simulink model "WTLV"  (R2023a)
settings: Solver=VariableStepAuto  StartTime=0.0  StopTime=5  RelTol=1e-3
values from neighbouring files (symbols this model uses):
  Cbus = 80e-3    (= 0.08)    [DFIG_init5.m]
  D = 1e-3    (= 0.001)    [DFIG_init5.m]
  f = 50    [DFIG_init5.m]
  Fs = Vs*sqrt(2/3)/(2*pi*f)    [DFIG_init5.m]
  fsw = 4e3    (= 4000)    [DFIG_init5.m]
  Is = 1760    [DFIG_init5.m]
  J = 127    [DFIG_init5.m]
  ki_id = (wni^2)*Lr*sigma    (= 491.599501999)    [DFIG_init5.m]
  ki_idg = (wnig^2)*Lg    (= 56.8489213503)    [DFIG_init5.m]
  ki_iq = ki_id    (= 491.599501999)    [DFIG_init5.m]
  ki_iqg = ki_idg    (= 56.8489213503)    [DFIG_init5.m]
  ki_n = (wnn^2)*J/p    (= 25400)    [DFIG_init5.m]
  ki_v = -300000    [DFIG_init5.m]
  Kopt = ((0.5*ro*pi* (Radio^5) *Cp_max)/(lambda_opt^3))    (= 296454.198186)    [DFIG_init5.m]
  kp_id = (2*wni*sigma*Lr)-Rr    (= 0.5771)    [DFIG_init5.m]
  kp_idg = (2*wnig*Lg)-Rg    (= 0.301572894745)    [DFIG_init5.m]
  kp_iq = kp_id    (= 0.5771)    [DFIG_init5.m]
  kp_iqg = kp_idg    (= 0.301572894745)    [DFIG_init5.m]
  kp_n = (2*wnn*J)/p    (= 2540)    [DFIG_init5.m]
  kp_v = -1000    [DFIG_init5.m]
  Kpg = 1/(1.5*Vs*sqrt(2/3))    [DFIG_init5.m]
  Kqg = -Kpg    [DFIG_init5.m]
  kT = -1.5*p*(Lm/Ls)*Fs    [DFIG_init5.m]
  Lg = 400e-6    (= 0.0004)    [DFIG_init5.m]
  Lm = 2.5e-3    (= 0.0025)    [DFIG_init5.m]
  Lr = Lm + Lsi    (= 0.002587)    [DFIG_init5.m]
  Ls = Lm + Lsi    (= 0.002587)    [DFIG_init5.m]
  Lsi = 0.087e-3    (= 8.7e-05)    [DFIG_init5.m]
  N = 100    [DFIG_init5.m]
  p = 2    [DFIG_init5.m]
  Ps = 2e6    (= 2000000)    [DFIG_init5.m]
  Radio = 42    [DFIG_init5.m]
  Rcrowbar = 0.2    [DFIG_init5.m]
  Rg = 20e-6    (= 2e-05)    [DFIG_init5.m]
  ro = 1.225    [DFIG_init5.m]
  Rr = 2.9e-3    (= 0.0029)    [DFIG_init5.m]
  Rs = 2.6e-3    (= 0.0026)    [DFIG_init5.m]
  sigma = 1-Lm^2/(Ls*Lr)    (= 0.0661284179513)    [DFIG_init5.m]
  smax = 1/3    (= 0.333333333333)    [DFIG_init5.m]
  t_dip = 3    [DFIG_init5.m]
  t_normal = 4.17    [DFIG_init5.m]
  t_recover = 3.5    [DFIG_init5.m]
  tab_lambda = [0.1:0.01:11.8]    [DFIG_init5.m]
  Tcrowbar = 0.1    [DFIG_init5.m]
  Tem = 12732    [DFIG_init5.m]
  Ts = 1/fsw/50    (= 5e-06)    [DFIG_init5.m]
  Vbus = 1150    [DFIG_init5.m]
  Vs = 690    [DFIG_init5.m]
undefined symbols (not defined in the file or in its folder): Ct, DiscIntNeverNeededParam
libraries: spsSeriesRLCBranchLib x5, spsUniversalBridgeLib x3, spsThreePhaseVIMeasurementLib x3, spsPWMGenerator2LevelLib x2, spsAsynchronousMachineSIUnitsLib x1, spsGroundLib x1, spsIdealSwitchLib x1, spsThreePhaseProgrammableVoltageSourceLib x1, spsThreePhaseTransformerTwoWindingsLib x1, spsEdgeDetectorLib x1, eeGeneralControl x1, sps_lib x1
settings Model: SimulationMode=accelerator  Creator=Qingyuan  LastModifiedBy=User
settings OptimizationCC: ReuseModelBlockBuffer=off

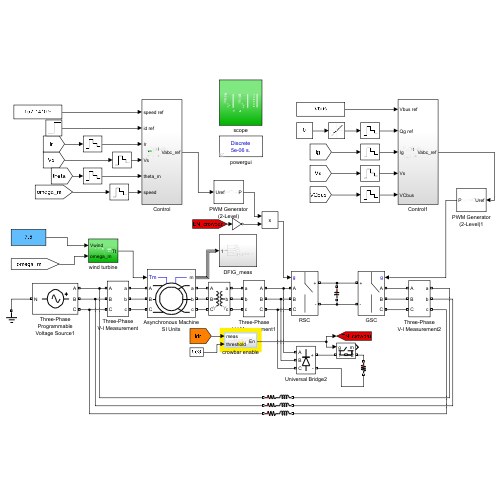
[thumbnail: Simulink's stored preview of the top-level diagram]
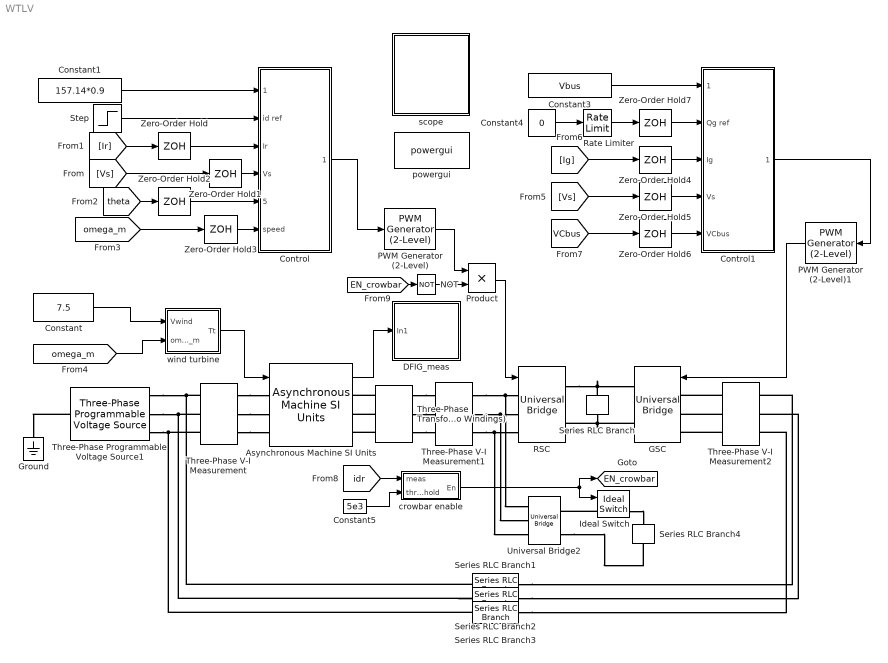
== system WTLV ==
  Asynchronous Machine SI Units : spsAsynchronousMachineSIUnitsLib/Asynchronous Machine SI Units  RotorType=Wound  PresetModel=No  MechanicalLoad=Torque Tm  ShowDetailedParameters=on  ReferenceFrame=Rotor  Units=SI  MeasurementBus=off  NominalParameters=[Ps Vs f]  VoltageRatio=1  Stator=[Rs Lsi]  Rotor=[Rr Lsi]  Cage1=[0.4155 0.002066]  Cage2=[0.4168 0.0003495]  Lm=Lm  Mechanical=[J D p]  PolePairs=2  InitialConditions=[1 0 0 0 0 0 0 0]  SimulateSaturation=off  Saturation=[14.03593122, 27.81365428, 53.79336849, 72.68890987, 97.98006896, 148.6815601, 215.7428561, 302.9841135, 428.7778367 ; 230, 322, 414, 460, 506, 552, 598, 644, 690]  LoadFlowParameters=1492000  TsPowergui=0  TsBlock=-1  IterativeModel=Trapezoidal non iterative  IterativeDiscreteModel=Trapezoidal non iterative  Pmec=1.4e6
  Constant : Constant  Value=7.5
  Constant1 : Constant  Value=157.14*0.9
  Constant3 : Constant  Value=Vbus
  Constant4 : Constant  Value=0
  Constant5 : Constant  Value=5e3
  Control : Subsystem
  Control1 : Subsystem
  DFIG_meas : Subsystem
  GSC : spsUniversalBridgeLib/Universal Bridge  Arms=3  SnubberResistance=1e5  SnubberCapacitance=inf  Device=Ideal Switches  Ron=1e-3  Lon=0  ForwardVoltages="[  0  0  ]"  ForwardVoltage=0  GTOparameters=[ 10e-6 , 20e-6 ]  IGBTparameters=[ 1e-6 , 2e-6 ]  Measurements=None  Measurements_2=None  converterType=Rectifier
  Ground : spsGroundLib/Ground  LConnTagsString=a
  Ideal Switch : spsIdealSwitchLib/Ideal Switch  Ron=0.001  Lon=0  IC=0  Rs=1e5  Cs=inf  Measurements=on
  NOT : Logic  Operator=NOT  IconShape=distinctive  AllPortsSameDT=off  OutDataTypeStr=boolean
  PWM Generator (2-Level) : spsPWMGenerator2LevelLib/PWM Generator (2-Level)  ModulatorType=Three-phase bridge (6 pulses)  ModulatorMode=Unsynchronized  Fc=fsw  Pc=0  nF=27  MinMax="[ -1  1 ]"  SamplingTechnique=Symmetrical regular (single edge)  ModulatingSignals=off  m=0.8  Freq=60  Phase=0  Ts=0  ShowCarrierOutport=off
  PWM Generator (2-Level)1 : spsPWMGenerator2LevelLib/PWM Generator (2-Level)  ModulatorType=Three-phase bridge (6 pulses)  ModulatorMode=Unsynchronized  Fc=fsw  Pc=0  nF=27  MinMax="[ -1  1 ]"  SamplingTechnique=Symmetrical regular (single edge)  ModulatingSignals=off  m=0.8  Freq=60  Phase=0  Ts=0  ShowCarrierOutport=off
  Product : Product
  RSC : spsUniversalBridgeLib/Universal Bridge  Arms=3  SnubberResistance=1e5  SnubberCapacitance=inf  Device=Ideal Switches  Ron=1e-3  Lon=0  ForwardVoltages="[  0  0  ]"  ForwardVoltage=0  GTOparameters=[ 10e-6 , 20e-6 ]  IGBTparameters=[ 1e-6 , 2e-6 ]  Measurements=None  Measurements_2=None  converterType=Rectifier
  Rate Limiter : RateLimiter  RisingSlewLimit=200e3  FallingSlewLimit=-200e3  SampleTimeMode=inherited
  Series RLC Branch : spsSeriesRLCBranchLib/Series RLC Branch  LConnTagsString=__new0  RConnTagsString=__new0  BranchType=C  Resistance=1  Inductance=1e-3  SetiL0=off  InitialCurrent=0  Capacitance=Cbus  Setx0=off  InitialVoltage=0  Measurements=Branch voltage
  Series RLC Branch1 : spsSeriesRLCBranchLib/Series RLC Branch  LConnTagsString=__new0  RConnTagsString=__new0  BranchType=RL  Resistance=Rg  Inductance=Lg  SetiL0=off  InitialCurrent=0  Capacitance=1e-6  Setx0=off  InitialVoltage=0  Measurements=None
  Series RLC Branch2 : spsSeriesRLCBranchLib/Series RLC Branch  LConnTagsString=__new0  RConnTagsString=__new0  BranchType=RL  Resistance=Rg  Inductance=Lg  SetiL0=off  InitialCurrent=0  Capacitance=1e-6  Setx0=off  InitialVoltage=0  Measurements=None
  Series RLC Branch3 : spsSeriesRLCBranchLib/Series RLC Branch  LConnTagsString=__new0  RConnTagsString=__new0  BranchType=RL  Resistance=Rg  Inductance=Lg  SetiL0=off  InitialCurrent=0  Capacitance=1e-6  Setx0=off  InitialVoltage=0  Measurements=None
  Series RLC Branch4 : spsSeriesRLCBranchLib/Series RLC Branch  LConnTagsString=__new0  RConnTagsString=__new0  BranchType=R  Resistance=Rcrowbar  Inductance=1e-3  SetiL0=off  InitialCurrent=0  Capacitance=Cbus  Setx0=off  InitialVoltage=0  Measurements=Branch current
  Step : Step  Time=t_dip+0.1  After=Is  SampleTime=0
  Three-Phase Programmable Voltage Source1 : spsThreePhaseProgrammableVoltageSourceLib/Three-Phase Programmable Voltage Source  PositiveSequence="[Vs*0.1  0 f]"  VariationEntity=Amplitude  VariationType=Ramp  VariationTypeAlt=Step  VariationStep=0.5  VariationRate=15  VariationMagnitude=0.3  VariationFrequency=2  VariationTiming=[t_recover t_normal]  VariationPhaseA=off  Amplitudes=[1 0.8 1.2 1.0]  TimeValues=[0 0.1 0.15 0.2]  HarmonicGeneration=on  HarmonicA=[1 10 0 1]  HarmonicB=[0 0 0 0]  Timing="[0  t_dip]"  BusType=swing  Pref=0  Qref=0  Qmin=-inf  Qmax=inf
  Three-Phase Transformer (Two Windings) : spsThreePhaseTransformerTwoWindingsLib/Three-Phase Transformer (Two Windings)  Winding1Connection=Y  Winding2Connection=Y  CoreType=Three single-phase transformers  SetSaturation=off  Hysteresis=off  DataFile='hysteresis'  SetInitialFlux=off  Measurements=None  UNITS=SI  NominalPower=[ Ps , f ]  Winding1=[Vs 0 0]  Winding2=[Vs/u 0 0]  Rm=1.3506e+08  Lm=4.299e+05  L0=0.5  Saturation=[0 0;0.0053322 2292.3;2.2218 2903.6]  InitialFluxes=[ 0.8 , -0.8 , 0.7 ]  BreakLoop=off  DiscreteSolver=Trapezoidal iterative  DataType=on  TransfoNumber=1
  Three-Phase V-I Measurement : spsThreePhaseVIMeasurementLib/Three-Phase V-I Measurement  VoltageMeasurement=phase-to-ground  SetLabelV=on  LabelV=Vs  Vpu=off  VpuLL=off  CurrentMeasurement=yes  SetLabelI=on  LabelI=Is  Ipu=off  Pbase=100e6  Vbase=500e3  OutputType=Complex  PhasorSimulation=off  PSBequivalent=0
  Three-Phase V-I Measurement1 : spsThreePhaseVIMeasurementLib/Three-Phase V-I Measurement  VoltageMeasurement=no  SetLabelV=off  LabelV=Vc  Vpu=off  VpuLL=off  CurrentMeasurement=yes  SetLabelI=on  LabelI=Ir  Ipu=off  Pbase=100e6  Vbase=500e3  OutputType=Complex  PhasorSimulation=off  PSBequivalent=0
  Three-Phase V-I Measurement2 : spsThreePhaseVIMeasurementLib/Three-Phase V-I Measurement  VoltageMeasurement=no  SetLabelV=off  LabelV=Vc  Vpu=off  VpuLL=off  CurrentMeasurement=yes  SetLabelI=on  LabelI=Ig  Ipu=off  Pbase=100e6  Vbase=500e3  OutputType=Complex  PhasorSimulation=off  PSBequivalent=0
  Universal Bridge2 : spsUniversalBridgeLib/Universal Bridge  Arms=3  SnubberResistance=1e5  SnubberCapacitance=inf  Device=Diodes  Ron=1e-3  Lon=0  ForwardVoltages="[  0  0  ]"  ForwardVoltage=0  GTOparameters=[ 10e-6 , 20e-6 ]  IGBTparameters=[ 1e-6 , 2e-6 ]  Measurements=None  Measurements_2=None  converterType=Rectifier
  Zero-Order Hold{,1..7} (8 alike) : ZeroOrderHold  SampleTime=1/fsw
  crowbar enable : Subsystem
  powergui : sps_lib/powergui  Priority=1  SimulationMode=Discrete  SampleTime=Ts  frequency=60  Iterations=50  frequencyindice=50  Pbase=100e6  ErrMax=1e-4  UnitsV=kV  UnitsW=MW  buscounter=0  FunctionMessages=off  echomessages=off  EnableUseOfTLC=off  CurrentSourceSwitches=off  DisableSnubberDevices=off  DisableRonSwitches=off  DisableVfSwitches=off  DisplayEquations=off  AutomaticDiscreteSolvers=off  SolverType=Tustin/Backward Euler (TBE)  Interpol=off  ExternalGateDelay=off  methode=off  Ts=100  x0status=blocks  SPID=on  SwTol=0  HookPort=off  NonlinearTolerance=1e-4  nMaxIteration=100  ContinueOnMaxIteration=off  RestoreLinks=warning  ResistiveCurrentMeasurement=off  Frange=[0:2:500]  Ylog=off  Xlog=on  ShowGrid=off  save=off  variable=ZData  structure=0  ZoomFFT=off  StartTime=0.0  cycles=1  DisplayStyle=1  fundamental=60  FreqAxis=off  MaxFrequency=1000  frequencyindicesteady=1  RmsSteady=1  display=off
  scope : Subsystem
  wind turbine : Subsystem
  tag scope: EN_crowbar=global
  wires:
  Control/1(Vabc_ref) -> PWM Generator (2-Level)/1
  [Vs] -> Zero-Order Hold1/1
  [Ir] -> Zero-Order Hold/1
  Constant1/1 -> Control/1(speed ref)
  Step/1 -> Control/2(id ref)
  [theta] -> Zero-Order Hold2/1
  [omega_m] -> Zero-Order Hold3/1
  Asynchronous Machine SI Units/1 -> DFIG_meas/1(In1)
  Zero-Order Hold/1 -> Control/3(Ir)
  Zero-Order Hold1/1 -> Control/4(Vs)
  Zero-Order Hold2/1 -> Control/5(theta_m)
  Zero-Order Hold3/1 -> Control/6(speed)
  Constant/1 -> wind turbine/1(Vwind)
  wind turbine/1(Tt) -> Asynchronous Machine SI Units/1
  [omega_m] -> wind turbine/2(omega_m)
  Zero-Order Hold5/1 -> Control1/4(Vs)
  Zero-Order Hold4/1 -> Control1/3(Ig)
  Constant4/1 -> Rate Limiter/1
  Constant3/1 -> Control1/1(Vbus ref)
  [Ig] -> Zero-Order Hold4/1
  [Vs] -> Zero-Order Hold5/1
  Control1/1(Vabc_ref) -> PWM Generator (2-Level)1/1
  [VCbus] -> Zero-Order Hold6/1
  Zero-Order Hold6/1 -> Control1/5(VCbus)
  Rate Limiter/1 -> Zero-Order Hold7/1
  Zero-Order Hold7/1 -> Control1/2(Qg ref)
  Constant5/1 -> crowbar enable/2(threshold)
  crowbar enable/1(En) -> Ideal Switch/1, [EN_crowbar]
  [idr] -> crowbar enable/1(meas)
  NOT/1 -> Product/2
  [EN_crowbar] -> NOT/1
  PWM Generator (2-Level)1/1 -> GSC/1
  PWM Generator (2-Level)/1 -> Product/1
  Product/1 -> RSC/1
  connections:
  Three-Phase Programmable Voltage Source1/LConn1 -- Ground/LConn1
  Three-Phase V-I Measurement/LConn1 -- Three-Phase Programmable Voltage Source1/RConn1 -- Series RLC Branch1/LConn1
  Three-Phase V-I Measurement/LConn2 -- Three-Phase Programmable Voltage Source1/RConn2 -- Series RLC Branch2/LConn1
  Three-Phase V-I Measurement/LConn3 -- Series RLC Branch3/LConn1 -- Three-Phase Programmable Voltage Source1/RConn3
  Three-Phase V-I Measurement/RConn1 -- Asynchronous Machine SI Units/LConn1
  Three-Phase V-I Measurement/RConn2 -- Asynchronous Machine SI Units/LConn2
  Three-Phase V-I Measurement/RConn3 -- Asynchronous Machine SI Units/LConn3
  Three-Phase V-I Measurement1/LConn1 -- Universal Bridge2/LConn1 -- RSC/LConn1
  Three-Phase V-I Measurement1/LConn3 -- Universal Bridge2/LConn3 -- RSC/LConn3
  Three-Phase V-I Measurement1/LConn2 -- Universal Bridge2/LConn2 -- RSC/LConn2
  Three-Phase Transformer (Two Windings)/RConn1 -- Three-Phase V-I Measurement1/RConn1
  Three-Phase Transformer (Two Windings)/RConn2 -- Three-Phase V-I Measurement1/RConn2
  Three-Phase Transformer (Two Windings)/RConn3 -- Three-Phase V-I Measurement1/RConn3
  RSC/RConn1 -- Series RLC Branch/LConn1 -- GSC/RConn1
  GSC/RConn2 -- RSC/RConn2 -- Series RLC Branch/RConn1
  Three-Phase V-I Measurement2/LConn1 -- GSC/LConn1
  Three-Phase V-I Measurement2/LConn2 -- GSC/LConn2
  Three-Phase V-I Measurement2/LConn3 -- GSC/LConn3
  Series RLC Branch1/RConn1 -- Three-Phase V-I Measurement2/RConn1
  Series RLC Branch2/RConn1 -- Three-Phase V-I Measurement2/RConn2
  Series RLC Branch3/RConn1 -- Three-Phase V-I Measurement2/RConn3
  Three-Phase Transformer (Two Windings)/LConn3 -- Asynchronous Machine SI Units/RConn3
  Three-Phase Transformer (Two Windings)/LConn2 -- Asynchronous Machine SI Units/RConn2
  Three-Phase Transformer (Two Windings)/LConn1 -- Asynchronous Machine SI Units/RConn1
  Ideal Switch/LConn1 -- Universal Bridge2/RConn1
  Ideal Switch/RConn1 -- Series RLC Branch4/LConn1
  Universal Bridge2/RConn2 -- Series RLC Branch4/RConn1

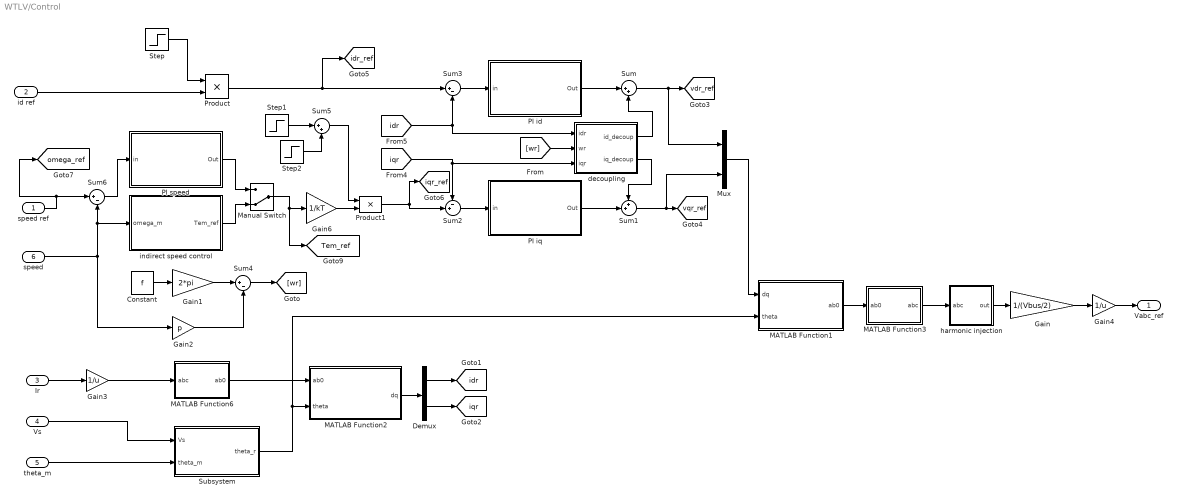
== system WTLV/Control ==
  speed ref : Inport
  id ref : Inport  Port=2
  Ir : Inport  Port=3
  Vs : Inport  Port=4
  theta_m : Inport  Port=5
  speed : Inport  Port=6
  Constant : Constant  Value=f
  Demux : Demux  Outputs=2
  Gain : Gain  Gain=1/(Vbus/2)
  Gain1 : Gain  Gain=2*pi
  Gain2 : Gain  Gain=p
  Gain3 : Gain  Gain=1/u
  Gain4 : Gain  Gain=1/u
  Gain6 : Gain  Gain=1/kT
  MATLAB Function1 : MATLAB Function  TreatAsAtomicUnit=on
  MATLAB Function2 : MATLAB Function  TreatAsAtomicUnit=on
  MATLAB Function3 : MATLAB Function  TreatAsAtomicUnit=on
  MATLAB Function6 : MATLAB Function  TreatAsAtomicUnit=on
  Manual Switch : ManualSwitch  CurrentSetting=0
  Mux : Mux  Inputs=2
  PI id : Subsystem
  PI iq : Subsystem
  PI speed : Subsystem
  Product : Product
  Product1 : Product
  Step : Step  Time=t_normal  Before=1  After=0  SampleTime=0
  Step1 : Step  Time=t_dip+0.15  Before=1  After=0  SampleTime=0
  Step2 : Step  Time=t_normal  SampleTime=0
  Subsystem : Subsystem
  Sum : Sum  Inputs=|++
  Sum1 : Sum  Inputs=++|
  Sum2 : Sum  Inputs=-+|
  Sum3 : Sum  Inputs=|+-
  Sum4 : Sum  Inputs=|+-
  Sum5 : Sum  Inputs=|++
  Sum6 : Sum  Inputs=|+-
  decoupling : Subsystem
  harmonic injection : Subsystem
  indirect speed control : Subsystem
  Vabc_ref : Outport
  tag scope: Tem_ref=global, idr=global, idr_ref=global, iqr=global, iqr_ref=global, omega_ref=global, vdr_ref=global, vqr_ref=global
  wires:
  MATLAB Function3/1(abc) -> harmonic injection/1(abc)
  MATLAB Function1/1(ab0) -> MATLAB Function3/1(ab0)
  Gain/1 -> Gain4/1
  harmonic injection/1(out) -> Gain/1
  Vs/1 -> Subsystem/1(Vs)
  theta_m/1 -> Subsystem/2(theta_m)
  MATLAB Function6/1(ab0) -> MATLAB Function2/1(ab0)
  Ir/1 -> Gain3/1
  Subsystem/1(theta_r) -> MATLAB Function1/2(theta), MATLAB Function2/2(theta)
  Sum2/1 -> PI iq/1(in)
  Sum3/1 -> PI id/1(in)
  Constant/1 -> Gain1/1
  Gain1/1 -> Sum4/1
  Gain2/1 -> Sum4/2
  Sum4/1 -> [wr]
  MATLAB Function2/1(dq) -> Demux/1
  Demux/2 -> [iqr]
  Demux/1 -> [idr]
  Sum/1 -> Mux/1, [vdr_ref]
  Sum1/1 -> [vqr_ref], Mux/2
  Mux/1 -> MATLAB Function1/1(dq)
  Sum6/1 -> PI speed/1(in)
  speed ref/1 -> [omega_ref], Sum6/1
  Product/1 -> [idr_ref], Sum3/1
  Product1/1 -> [iqr_ref], Sum2/2
  [idr] -> Sum3/2, decoupling/1(idr)
  PI id/1(Out) -> Sum/1
  decoupling/1(id_decoup) -> Sum/2
  PI iq/1(Out) -> Sum1/2
  decoupling/2(iq_decoup) -> Sum1/1
  [iqr] -> Sum2/1, decoupling/3(iqr)
  [wr] -> decoupling/2(wr)
  Manual Switch/1 -> [Tem_ref], Gain6/1
  PI speed/1(Out) -> Manual Switch/1
  indirect speed control/1(Tem_ref) -> Manual Switch/2
  speed/1 -> Gain2/1, indirect speed control/1(omega_m), Sum6/2
  Gain3/1 -> MATLAB Function6/1(abc)
  Gain4/1 -> Vabc_ref/1
  id ref/1 -> Product/2
  Step/1 -> Product/1
  Gain6/1 -> Product1/2
  Step1/1 -> Sum5/1
  Step2/1 -> Sum5/2
  Sum5/1 -> Product1/1

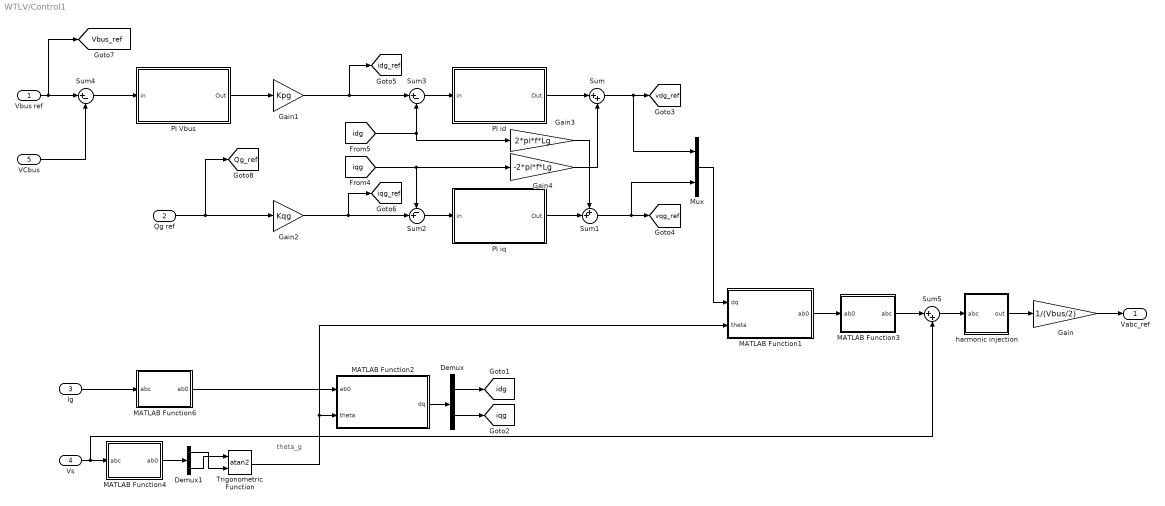
== system WTLV/Control1 ==
  note: theta_g
  Vbus ref : Inport
  Qg ref : Inport  Port=2
  Ig : Inport  Port=3
  Vs : Inport  Port=4
  VCbus : Inport  Port=5
  Demux : Demux  Outputs=2
  Demux1 : Demux  Outputs=2
  Gain : Gain  Gain=1/(Vbus/2)
  Gain1 : Gain  Gain=Kpg
  Gain2 : Gain  Gain=Kqg
  Gain3 : Gain  Gain=2*pi*f*Lg
  Gain4 : Gain  Gain=-2*pi*f*Lg
  MATLAB Function1 : MATLAB Function  TreatAsAtomicUnit=on
  MATLAB Function2 : MATLAB Function  TreatAsAtomicUnit=on
  MATLAB Function3 : MATLAB Function  TreatAsAtomicUnit=on
  MATLAB Function4 : MATLAB Function  TreatAsAtomicUnit=on
  MATLAB Function6 : MATLAB Function  TreatAsAtomicUnit=on
  Mux : Mux  Inputs=2
  PI Vbus : Subsystem
  PI id : Subsystem
  PI iq : Subsystem
  Sum : Sum  Inputs=|++
  Sum1 : Sum  Inputs=++|
  Sum2 : Sum  Inputs=-+|
  Sum3 : Sum  Inputs=|+-
  Sum4 : Sum  Inputs=|+-
  Sum5 : Sum  Inputs=|++
  Trigonometric Function : Trigonometry  Operator=atan2
  harmonic injection : Subsystem
  Vabc_ref : Outport
  tag scope: Qg_ref=global, Vbus_ref=global, idg=global, idg_ref=global, iqg=global, iqg_ref=global, vdg_ref=global, vqg_ref=global
  wires:
  PI Vbus/1(Out) -> Gain1/1
  [iqg] -> Sum2/1, Gain4/1
  Gain3/1 -> Sum1/1
  PI iq/1(Out) -> Sum1/2
  Gain4/1 -> Sum/2
  PI id/1(Out) -> Sum/1
  [idg] -> Gain3/1, Sum3/2
  Gain2/1 -> Sum2/2, [iqg_ref]
  Mux/1 -> MATLAB Function1/1(dq)
  Sum1/1 -> Mux/2, [vqg_ref]
  Sum/1 -> [vdg_ref], Mux/1
  Demux/1 -> [idg]
  Demux/2 -> [iqg]
  MATLAB Function2/1(dq) -> Demux/1
  Sum3/1 -> PI id/1(in)
  Sum2/1 -> PI iq/1(in)
  Trigonometric Function/1 -> MATLAB Function2/2(theta), MATLAB Function1/2(theta)
  Ig/1 -> MATLAB Function6/1(abc)
  MATLAB Function6/1(ab0) -> MATLAB Function2/1(ab0)
  Vs/1 -> Sum5/2, MATLAB Function4/1(abc)
  harmonic injection/1(out) -> Gain/1
  Gain/1 -> Vabc_ref/1
  MATLAB Function1/1(ab0) -> MATLAB Function3/1(ab0)
  MATLAB Function4/1(ab0) -> Demux1/1
  Demux1/1 -> Trigonometric Function/2
  Demux1/2 -> Trigonometric Function/1
  Gain1/1 -> [idg_ref], Sum3/1
  Qg ref/1 -> [Qg_ref], Gain2/1
  VCbus/1 -> Sum4/2
  Vbus ref/1 -> [Vbus_ref], Sum4/1
  Sum4/1 -> PI Vbus/1(in)
  Sum5/1 -> harmonic injection/1(abc)
  MATLAB Function3/1(abc) -> Sum5/1

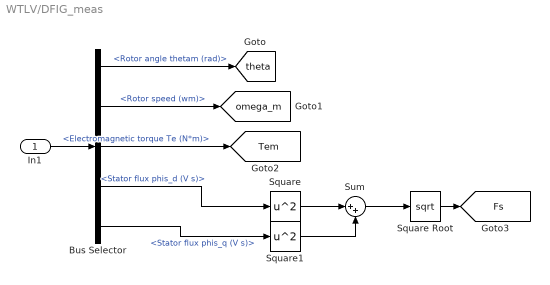
== system WTLV/DFIG_meas ==
  In1 : Inport
  Bus Selector : BusSelector  OutputSignals=Mechanical.Rotor angle thetam (rad),Mechanical.Rotor speed (wm),Mechanical.Electromagnetic torque Te (N*m),Stator measurements.Stator flux phis_d (V s),Stator measurements.Stator flux phis_q (V s)
  Square : Math  Operator=square
  Square Root : Sqrt
  Square1 : Math  Operator=square
  Sum : Sum  Inputs=|++
  tag scope: Fs=global, Tem=global, omega_m=global, theta=global
  wires:
  Bus Selector/1 -> [theta]  "<Rotor angle thetam (rad)>"
  Bus Selector/2 -> [omega_m]  "<Rotor speed (wm)>"
  In1/1 -> Bus Selector/1
  Bus Selector/3 -> [Tem]  "<Electromagnetic torque Te (N*m)>"
  Bus Selector/4 -> Square/1  "<Stator flux phis_d (V s)>"
  Bus Selector/5 -> Square1/1  "<Stator flux phis_q (V s)>"
  Square/1 -> Sum/1
  Sum/1 -> Square Root/1
  Square1/1 -> Sum/2
  Square Root/1 -> [Fs]

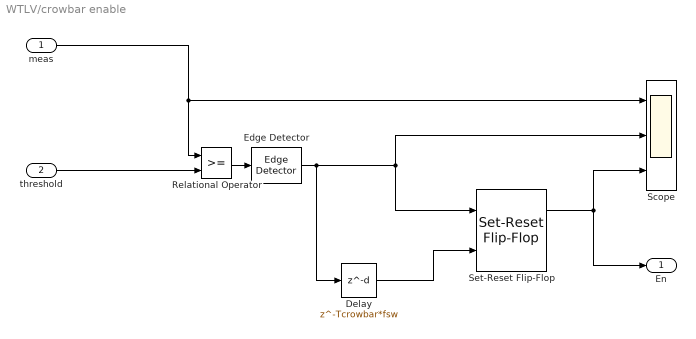
== system WTLV/crowbar enable ==
  meas : Inport
  threshold : Inport  Port=2
  Delay : Delay  DelayLength=Tcrowbar*fsw  SampleTime=1/fsw
  Edge Detector : spsEdgeDetectorLib/Edge Detector  model=Rising  ic=0  Ts=1/fsw
      settings: LibrarySourceBlock=sps_lib/Control/Edge Detector
  Relational Operator : RelationalOperator  OutDataTypeStr=boolean  RndMeth=Simplest  InputSameDT=off
  Scope : Scope  NumInputPorts=3
  Set-Reset Flip-Flop : eeGeneralControl/Set-Reset Flip-Flop  LabelModeActiveChoice=Discrete  UndefState=Set  Q0=0  Ts=0.5/fsw
      settings: LibrarySourceBlock=ee_sl_lib/General Control/Set-Reset Flip-Flop
  En : Outport
  wires:
  threshold/1 -> Relational Operator/2
  Relational Operator/1 -> Edge Detector/1
  meas/1 -> Scope/1, Relational Operator/1
  Edge Detector/1 -> Delay/1, Set-Reset Flip-Flop/1, Scope/2
  Delay/1 -> Set-Reset Flip-Flop/2
  Set-Reset Flip-Flop/1 -> En/1, Scope/3

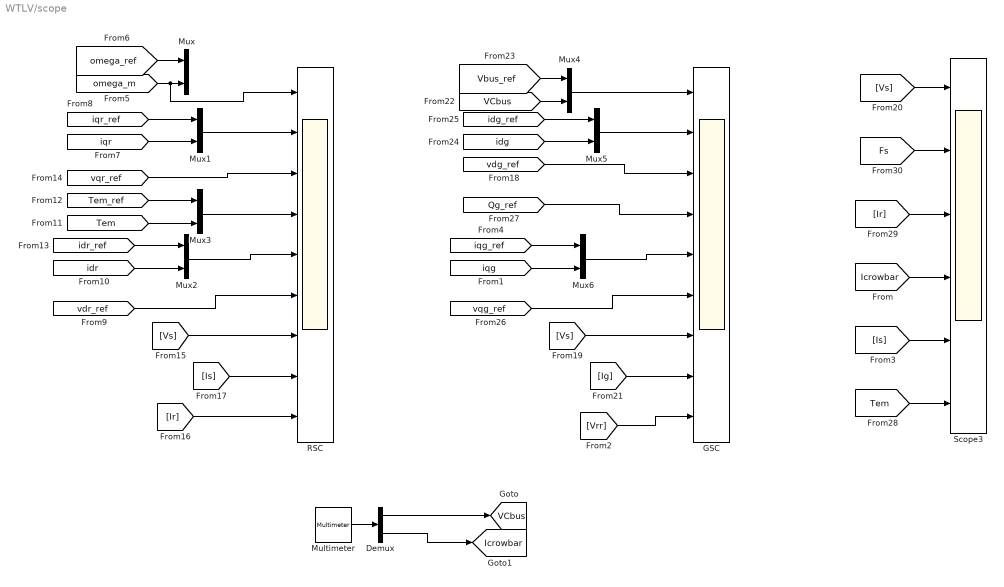
== system WTLV/scope ==
  Demux : Demux  Outputs=2
  GSC : Scope  NumInputPorts=9
  Multimeter : spsMultimeterLib/Multimeter  L=2  sel=[1 2]  yselected={}  Gain=[1 1]  OutputType=Complex  PlotAtSimulationStop=off  PhasorSimulation=off
  Mux{,1..6} (7 alike) : Mux  Inputs=2
  RSC : Scope  NumInputPorts=9
  Scope3 : Scope  NumInputPorts=6
  tag scope: Icrowbar=global, VCbus=global
  wires:
  [omega_ref] -> Mux/1
  [iqr] -> Mux1/2
  [omega_m] -> RSC/1, Mux/2
  [Vs] -> RSC/7
  [Tem] -> Mux3/2
  [Ir] -> RSC/9
  [Tem_ref] -> Mux3/1
  Mux1/1 -> RSC/2
  [idr] -> Mux2/2
  [vqr_ref] -> RSC/3
  [idr_ref] -> Mux2/1
  Mux3/1 -> RSC/4
  [iqr_ref] -> Mux1/1
  Mux2/1 -> RSC/5
  [vdr_ref] -> RSC/6
  [Is] -> RSC/8
  [Ig] -> GSC/8
  [vqg_ref] -> GSC/6
  Mux6/1 -> GSC/5
  [idg_ref] -> Mux5/1
  [iqg_ref] -> Mux6/1
  [vdg_ref] -> GSC/3
  [iqg] -> Mux6/2
  Mux5/1 -> GSC/2
  [Vs] -> GSC/7
  [VCbus] -> Mux4/2
  [idg] -> Mux5/2
  [Vbus_ref] -> Mux4/1
  Mux4/1 -> GSC/1
  [Qg_ref] -> GSC/4
  [Vrr] -> GSC/9
  Multimeter/1 -> Demux/1
  Demux/1 -> [VCbus]
  Demux/2 -> [Icrowbar]
  [Icrowbar] -> Scope3/4
  [Vs] -> Scope3/1
  [Is] -> Scope3/5
  [Tem] -> Scope3/6
  [Ir] -> Scope3/3
  [Fs] -> Scope3/2

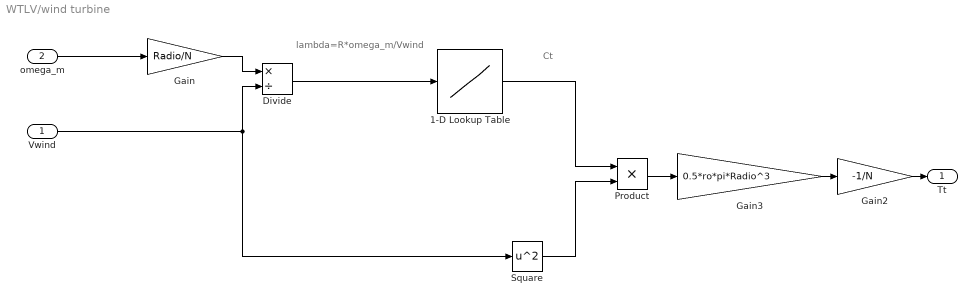
== system WTLV/wind turbine ==
  note: Ct
  note: lambda=R*omega_m/Vwind
  Vwind : Inport
  omega_m : Inport  Port=2
  1-D Lookup Table : Lookup_n-D  NumberOfTableDimensions=1  BreakpointsForDimension1=tab_lambda  Table=Ct  InternalRulePriority=Speed  RndMeth=Simplest
  Divide : Product  Inputs=*/
  Gain : Gain  Gain=Radio/N
  Gain2 : Gain  Gain=-1/N
  Gain3 : Gain  Gain=0.5*ro*pi*Radio^3
  Product : Product
  Square : Math  Operator=square
  Tt : Outport
  wires:
  Gain/1 -> Divide/1
  omega_m/1 -> Gain/1
  Vwind/1 -> Square/1, Divide/2
  Divide/1 -> 1-D Lookup Table/1
  Square/1 -> Product/2
  1-D Lookup Table/1 -> Product/1
  Product/1 -> Gain3/1
  Gain3/1 -> Gain2/1
  Gain2/1 -> Tt/1

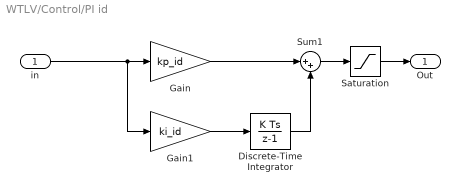
== system WTLV/Control/PI id ==
  in : Inport
  Discrete-Time Integrator : DiscreteIntegrator  SampleTime=1/fsw  LimitOutput=on  UpperSaturationLimit=Vbus/sqrt(3)  LowerSaturationLimit=-Vbus/sqrt(3)  ICPrevOutput=DiscIntNeverNeededParam  ICPrevScaledInput=DiscIntNeverNeededParam
  Gain : Gain  Gain=kp_id
  Gain1 : Gain  Gain=ki_id
  Saturation : Saturate  UpperLimit=Vbus/sqrt(3)  LowerLimit=-Vbus/sqrt(3)
  Sum1 : Sum  Inputs=|++
  Out : Outport
  wires:
  in/1 -> Gain1/1, Gain/1
  Gain1/1 -> Discrete-Time Integrator/1
  Gain/1 -> Sum1/1
  Discrete-Time Integrator/1 -> Sum1/2
  Sum1/1 -> Saturation/1
  Saturation/1 -> Out/1

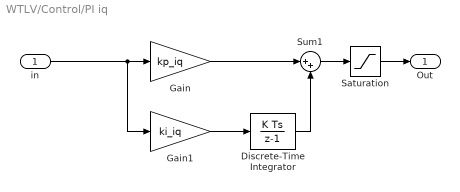
== system WTLV/Control/PI iq ==
  in : Inport
  Discrete-Time Integrator : DiscreteIntegrator  SampleTime=1/fsw  LimitOutput=on  UpperSaturationLimit=Vbus/sqrt(3)  LowerSaturationLimit=-Vbus/sqrt(3)  ICPrevOutput=DiscIntNeverNeededParam  ICPrevScaledInput=DiscIntNeverNeededParam
  Gain : Gain  Gain=kp_iq
  Gain1 : Gain  Gain=ki_iq
  Saturation : Saturate  UpperLimit=Vbus/sqrt(3)  LowerLimit=-Vbus/sqrt(3)
  Sum1 : Sum  Inputs=|++
  Out : Outport
  wires:
  Saturation/1 -> Out/1
  Sum1/1 -> Saturation/1
  Discrete-Time Integrator/1 -> Sum1/2
  Gain/1 -> Sum1/1
  Gain1/1 -> Discrete-Time Integrator/1
  in/1 -> Gain/1, Gain1/1

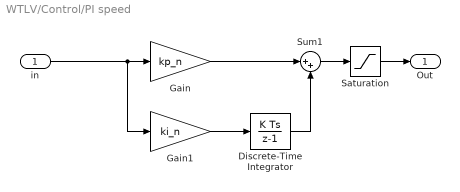
== system WTLV/Control/PI speed ==
  in : Inport
  Discrete-Time Integrator : DiscreteIntegrator  SampleTime=1/fsw  LimitOutput=on  UpperSaturationLimit=Tem  LowerSaturationLimit=-Tem  ICPrevOutput=DiscIntNeverNeededParam  ICPrevScaledInput=DiscIntNeverNeededParam
  Gain : Gain  Gain=kp_n
  Gain1 : Gain  Gain=ki_n
  Saturation : Saturate  UpperLimit=Tem  LowerLimit=-Tem
  Sum1 : Sum  Inputs=|++
  Out : Outport
  wires:
  Saturation/1 -> Out/1
  Sum1/1 -> Saturation/1
  Discrete-Time Integrator/1 -> Sum1/2
  Gain/1 -> Sum1/1
  Gain1/1 -> Discrete-Time Integrator/1
  in/1 -> Gain/1, Gain1/1

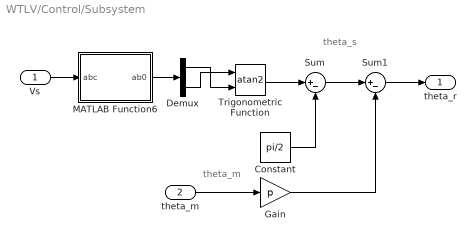
== system WTLV/Control/Subsystem ==
  note: theta_s
  note: theta_m
  Vs : Inport
  theta_m : Inport  Port=2
  Constant : Constant  Value=pi/2
  Demux : Demux  Outputs=2
  Gain : Gain  Gain=p
  MATLAB Function6 : MATLAB Function  TreatAsAtomicUnit=on
  Sum : Sum  Inputs=|+-
  Sum1 : Sum  Inputs=|+-
  Trigonometric Function : Trigonometry  Operator=atan2
  theta_r : Outport
  wires:
  Vs/1 -> MATLAB Function6/1(abc)
  theta_m/1 -> Gain/1
  MATLAB Function6/1(ab0) -> Demux/1
  Demux/1 -> Trigonometric Function/2
  Demux/2 -> Trigonometric Function/1
  Trigonometric Function/1 -> Sum/1
  Constant/1 -> Sum/2
  Sum/1 -> Sum1/1
  Sum1/1 -> theta_r/1
  Gain/1 -> Sum1/2

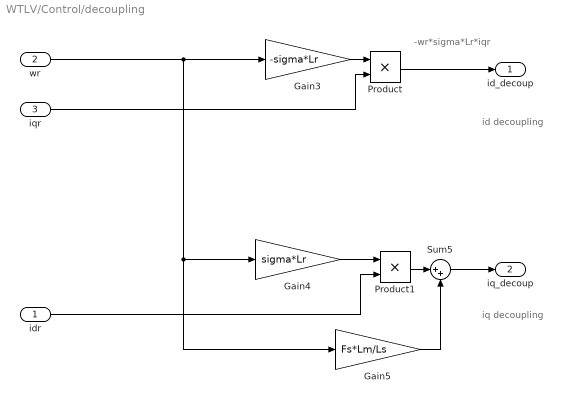
== system WTLV/Control/decoupling ==
  note: -wr*sigma*Lr*iqr
  note: id decoupling
  note: iq decoupling
  idr : Inport
  wr : Inport  Port=2
  iqr : Inport  Port=3
  Gain3 : Gain  Gain=-sigma*Lr
  Gain4 : Gain  Gain=sigma*Lr
  Gain5 : Gain  Gain=Fs*Lm/Ls
  Product : Product
  Product1 : Product
  Sum5 : Sum  Inputs=|++
  id_decoup : Outport
  iq_decoup : Outport  Port=2
  wires:
  Product1/1 -> Sum5/1
  wr/1 -> Gain5/1, Gain4/1, Gain3/1
  Sum5/1 -> iq_decoup/1
  Gain3/1 -> Product/1
  Gain4/1 -> Product1/1
  Gain5/1 -> Sum5/2
  iqr/1 -> Product/2
  idr/1 -> Product1/2
  Product/1 -> id_decoup/1

== system WTLV/Control/harmonic injection ==
  abc : Inport
  Gain : Gain  Gain=-0.5
  Min : MinMax
  Min1 : MinMax  Function=max
  Sum : Sum  Inputs=|++
  Sum1 : Sum  Inputs=|++
  out : Outport
  wires:
  Min/1 -> Sum/1
  Min1/1 -> Sum/2
  Sum1/1 -> out/1
  Sum/1 -> Gain/1
  abc/1 -> Min1/1, Min/1, Sum1/1
  Gain/1 -> Sum1/2

== system WTLV/Control/indirect speed control ==
  omega_m : Inport
  Gain : Gain  Gain=1/N
  Gain1 : Gain  Gain=-Kopt
  Gain2 : Gain  Gain=1/N
  Square : Math  Operator=square
  Tem_ref : Outport
  wires:
  omega_m/1 -> Gain/1
  Gain/1 -> Square/1
  Gain2/1 -> Tem_ref/1
  Square/1 -> Gain1/1
  Gain1/1 -> Gain2/1

== system WTLV/Control1/PI Vbus ==
  in : Inport
  Discrete-Time Integrator : DiscreteIntegrator  SampleTime=1/fsw  LimitOutput=on  UpperSaturationLimit=Ps*smax  LowerSaturationLimit=-Ps*smax  ICPrevOutput=DiscIntNeverNeededParam  ICPrevScaledInput=DiscIntNeverNeededParam
  Gain : Gain  Gain=kp_v
  Gain1 : Gain  Gain=ki_v
  Saturation : Saturate  UpperLimit=Ps*smax  LowerLimit=-Ps*smax
  Sum1 : Sum  Inputs=|++
  Out : Outport
  wires:
  in/1 -> Gain1/1, Gain/1
  Gain1/1 -> Discrete-Time Integrator/1
  Gain/1 -> Sum1/1
  Discrete-Time Integrator/1 -> Sum1/2
  Sum1/1 -> Saturation/1
  Saturation/1 -> Out/1

== system WTLV/Control1/PI id ==
  in : Inport
  Discrete-Time Integrator : DiscreteIntegrator  SampleTime=1/fsw  LimitOutput=on  UpperSaturationLimit=Vbus*sqrt(3)  LowerSaturationLimit=-Vbus/sqrt(3)  ICPrevOutput=DiscIntNeverNeededParam  ICPrevScaledInput=DiscIntNeverNeededParam
  Gain : Gain  Gain=kp_idg
  Gain1 : Gain  Gain=ki_idg
  Saturation : Saturate  UpperLimit=Vbus/sqrt(3)  LowerLimit=-Vbus/sqrt(3)
  Sum1 : Sum  Inputs=|++
  Out : Outport
  wires:
  Saturation/1 -> Out/1
  Sum1/1 -> Saturation/1
  Discrete-Time Integrator/1 -> Sum1/2
  Gain/1 -> Sum1/1
  Gain1/1 -> Discrete-Time Integrator/1
  in/1 -> Gain/1, Gain1/1

== system WTLV/Control1/PI iq ==
  in : Inport
  Discrete-Time Integrator : DiscreteIntegrator  SampleTime=1/fsw  LimitOutput=on  UpperSaturationLimit=Vbus/sqrt(3)  LowerSaturationLimit=-Vbus/sqrt(3)  ICPrevOutput=DiscIntNeverNeededParam  ICPrevScaledInput=DiscIntNeverNeededParam
  Gain : Gain  Gain=kp_iqg
  Gain1 : Gain  Gain=ki_iqg
  Saturation : Saturate  UpperLimit=Vbus/sqrt(3)  LowerLimit=-Vbus/sqrt(3)
  Sum1 : Sum  Inputs=|++
  Out : Outport
  wires:
  in/1 -> Gain1/1, Gain/1
  Gain1/1 -> Discrete-Time Integrator/1
  Gain/1 -> Sum1/1
  Discrete-Time Integrator/1 -> Sum1/2
  Sum1/1 -> Saturation/1
  Saturation/1 -> Out/1

== system WTLV/Control1/harmonic injection ==
  abc : Inport
  Gain : Gain  Gain=-0.5
  Min : MinMax
  Min1 : MinMax  Function=max
  Sum : Sum  Inputs=|++
  Sum1 : Sum  Inputs=|++
  out : Outport
  wires:
  Gain/1 -> Sum1/2
  abc/1 -> Sum1/1, Min/1, Min1/1
  Sum/1 -> Gain/1
  Sum1/1 -> out/1
  Min1/1 -> Sum/2
  Min/1 -> Sum/1

== matlab function WTLV/Control/MATLAB Function3 ==
  data: ab0 input; abc output
function abc = ab0_to_abc(ab0)
abc = zeros(3,1);
abc(1) = ab0(1);
abc(2) = -1/2 * ab0(1) + sqrt(3)/2 * ab0(2);
abc(3) = -1/2 * ab0(1) - sqrt(3)/2 * ab0(2);
end

== matlab function WTLV/Control/Subsystem/MATLAB Function6 ==
  data: abc input; ab0 output
function ab0 = abc_to_ab0(abc)
ab0 = zeros(2,1);
ab0(1) = 2/3 * (abc(1) - abc(2)/2 - abc(3)/2);
ab0(2) = 2/3 * ( (sqrt(3)/2)*abc(2) - (sqrt(3)/2)*abc(3));
end

== matlab function WTLV/Control/MATLAB Function2 ==
  data: ab0 input; dq output; theta input
function dq = ab0_to_dq(ab0, theta)
dq = zeros(2,1);
dq(1) = cos(theta)*ab0(1) + sin(theta)*ab0(2);
dq(2) = -sin(theta)*ab0(1) + cos(theta)*ab0(2);
end

== matlab function WTLV/Control1/MATLAB Function1 ==
  data: dq input; ab0 output; theta input
function ab0 = dq_to_ab0(dq, theta)
ab0 = zeros(2,1);
ab0(1) = dq(1) * cos(theta) - dq(2) * sin(theta);
ab0(2) = dq(1) * sin(theta) + dq(2) * cos(theta);

end

== matlab function WTLV/Control1/MATLAB Function2 ==
  data: ab0 input; dq output; theta input
function dq = ab0_to_dq(ab0, theta)
dq = zeros(2,1);
dq(1) = cos(theta)*ab0(1) + sin(theta)*ab0(2);
dq(2) = -sin(theta)*ab0(1) + cos(theta)*ab0(2);
end

== matlab function WTLV/Control1/MATLAB Function3 ==
  data: ab0 input; abc output
function abc = ab0_to_abc(ab0)
abc = zeros(3,1);
abc(1) = ab0(1);
abc(2) = -1/2 * ab0(1) + sqrt(3)/2 * ab0(2);
abc(3) = -1/2 * ab0(1) - sqrt(3)/2 * ab0(2);
end

== matlab function WTLV/Control/MATLAB Function6 ==
  data: abc input; ab0 output
function ab0 = abc_to_ab0(abc)
ab0 = zeros(2,1);
ab0(1) = 2/3 * (abc(1) - abc(2)/2 - abc(3)/2);
ab0(2) = 2/3 * ( (sqrt(3)/2)*abc(2) - (sqrt(3)/2)*abc(3));
end

== matlab function WTLV/Control1/MATLAB Function6 ==
  data: abc input; ab0 output
function ab0 = abc_to_ab0(abc)
ab0 = zeros(2,1);
ab0(1) = 2/3 * (abc(1) - abc(2)/2 - abc(3)/2);
ab0(2) = 2/3 * ( (sqrt(3)/2)*abc(2) - (sqrt(3)/2)*abc(3));
end

== matlab function WTLV/Control1/MATLAB Function4 ==
  data: abc input; ab0 output
function ab0 = abc_to_ab0(abc)
ab0 = zeros(2,1);
ab0(1) = 2/3 * (abc(1) - abc(2)/2 - abc(3)/2);
ab0(2) = 2/3 * ( (sqrt(3)/2)*abc(2) - (sqrt(3)/2)*abc(3));
end

== matlab function WTLV/Control/MATLAB Function1 ==
  data: dq input; ab0 output; theta input
function ab0 = dq_to_ab0(dq, theta)
ab0 = zeros(2,1);
ab0(1) = dq(1) * cos(theta) - dq(2) * sin(theta);
ab0(2) = dq(1) * sin(theta) + dq(2) * cos(theta);

end
